simulink model "hw1_q1"  (R2021b)
settings: Solver=VariableStepAuto  StartTime=0.0  StopTime=20  RelTol=1e-6
undefined symbols (not defined in the file): A, B, C, K, K_, L, x0
settings Model: Creator=zpyang  LastModifiedBy=zpyang

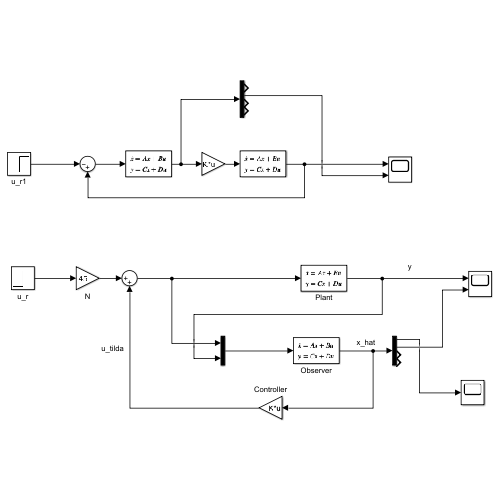
[thumbnail: Simulink's stored preview of the top-level diagram]
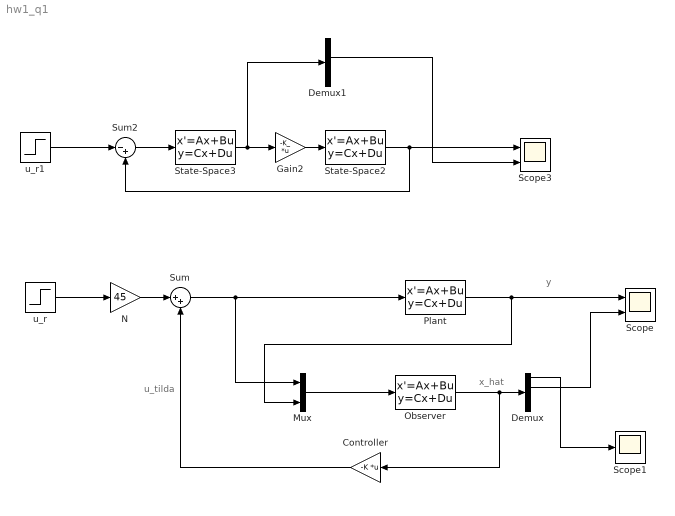
== system hw1_q1 ==
  note: u_tilda
  note: y
  note: x_hat
  Controller : Gain  Gain=-K  Multiplication=Matrix(K*u)
  Demux : Demux
  Demux1 : Demux
  Gain2 : Gain  Gain=-K_  Multiplication=Matrix(K*u)
  Mux : Mux  Inputs=2
  N : Gain  Gain=45
  Observer : StateSpace  A=A - L*C  B=[B L]  C=eye(4)  D=zeros(4,2)  InitialCondition=0
  Plant : StateSpace  A=A  B=B  C=C  D=0  InitialCondition=x0  ContinuousStateAttributes='state'
  Scope : Scope  NumInputPorts=2
  Scope1 : Scope
  Scope3 : Scope  NumInputPorts=2
  State-Space2 : StateSpace  A=A  B=B  C=C  D=0  InitialCondition=x0  ContinuousStateAttributes='state2'
  State-Space3 : StateSpace  A=A - B*K_ - L*C  B=L  C=eye(4)  D=zeros(4,1)  InitialCondition=0
  Sum : Sum  Inputs=|++
  Sum2 : Sum  Inputs=|-+
  u_r : Step  SampleTime=0
  u_r1 : Step  SampleTime=0
  wires:
  Plant/1 -> Mux/2, Scope/1
  Sum2/1 -> State-Space3/1
  State-Space2/1 -> Scope3/1, Sum2/2
  State-Space3/1 -> Demux1/1, Gain2/1
  Gain2/1 -> State-Space2/1
  u_r1/1 -> Sum2/1
  Sum/1 -> Mux/1, Plant/1
  Mux/1 -> Observer/1
  Observer/1 -> Controller/1, Demux/1
  Demux/2 -> Scope/2
  u_r/1 -> N/1
  Controller/1 -> Sum/2
  N/1 -> Sum/1
  Demux/1 -> Scope1/1
  Demux1/2 -> Scope3/2
